simulink model "threephase_transformer"  (R2021a)
settings: Solver=VariableStepAuto  StartTime=0.0  StopTime=0.05  RelTol=1e-3
libraries: spsCurrentMeasurementLib x6, spsVoltageMeasurementLib x6, spsACVoltageSourceLib x3, spsGroundLib x3, spsSeriesRLCBranchLib x3, spsThreePhaseTransformerTwoWindingsLib x1, spspowerguiLib x1
settings Model: Creator=Davie  LastModifiedBy=Davie

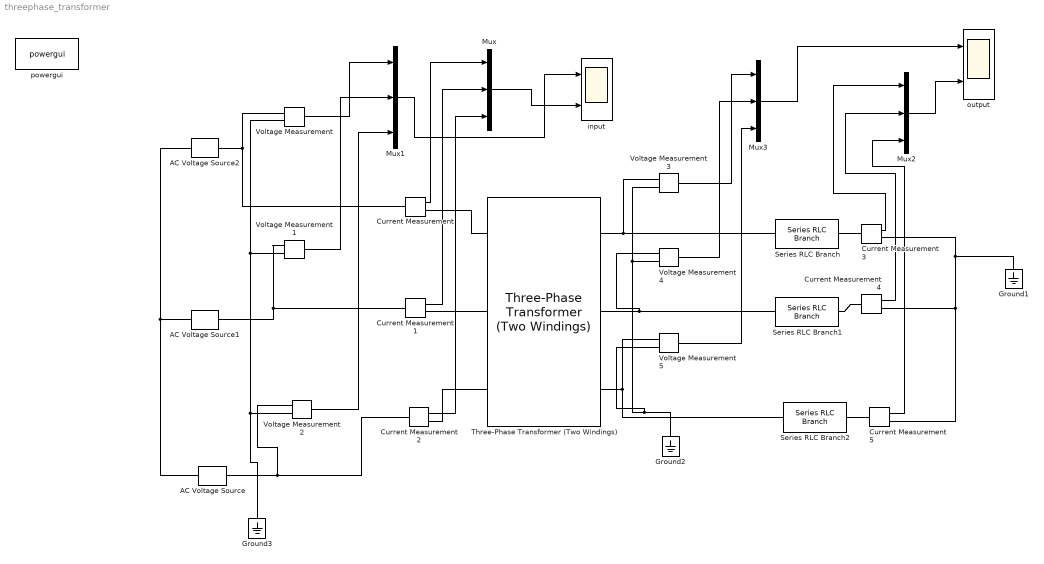
== system threephase_transformer ==
  AC Voltage Source : spsACVoltageSourceLib/AC Voltage Source  Amplitude=450  Phase=-120  Frequency=50  SampleTime=0  Measurements=None  BusType=swing  Pref=10e3  Qref=0  Qmin=-inf  Qmax=+inf
  AC Voltage Source1 : spsACVoltageSourceLib/AC Voltage Source  Amplitude=450  Phase=120  Frequency=50  SampleTime=0  Measurements=None  BusType=swing  Pref=10e3  Qref=0  Qmin=-inf  Qmax=+inf
  AC Voltage Source2 : spsACVoltageSourceLib/AC Voltage Source  Amplitude=450  Phase=0  Frequency=50  SampleTime=0  Measurements=None  BusType=swing  Pref=10e3  Qref=0  Qmin=-inf  Qmax=+inf
  Current Measurement{,1..5} (6 alike) : spsCurrentMeasurementLib/Current Measurement  PhasorSimulation=off  OutputType=Complex  PSBequivalent=0
  Ground1 : spsGroundLib/Ground  LConnTagsString=a
  Ground2 : spsGroundLib/Ground  LConnTagsString=a
  Ground3 : spsGroundLib/Ground  LConnTagsString=a
  Mux{,1..3} (4 alike) : Mux  Inputs=3
  Series RLC Branch : spsSeriesRLCBranchLib/Series RLC Branch  LConnTagsString=__new0  RConnTagsString=__new0  BranchType=R  Resistance=220  Inductance=1e-3  SetiL0=off  InitialCurrent=0  Capacitance=1e-6  Setx0=off  InitialVoltage=0  Measurements=None
  Series RLC Branch1 : spsSeriesRLCBranchLib/Series RLC Branch  LConnTagsString=__new0  RConnTagsString=__new0  BranchType=R  Resistance=220  Inductance=1e-3  SetiL0=off  InitialCurrent=0  Capacitance=1e-6  Setx0=off  InitialVoltage=0  Measurements=None
  Series RLC Branch2 : spsSeriesRLCBranchLib/Series RLC Branch  LConnTagsString=__new0  RConnTagsString=__new0  BranchType=R  Resistance=220  Inductance=1e-3  SetiL0=off  InitialCurrent=0  Capacitance=1e-6  Setx0=off  InitialVoltage=0  Measurements=None
  Three-Phase Transformer (Two Windings) : spsThreePhaseTransformerTwoWindingsLib/Three-Phase Transformer (Two Windings)  Winding1Connection=Yg  Winding2Connection=Yg  CoreType=Three single-phase transformers  SetSaturation=off  Hysteresis=off  DataFile='hysteresis'  SetInitialFlux=off  Measurements=None  UNITS=pu  NominalPower=[ 250e6 , 60 ]  Winding1=[ 440e3 , 0.002 , 0.08 ]  Winding2=[ 315e3 , 0.002 , 0.08 ]  Rm=500  Lm=500  L0=0.5  Saturation=[ 0,0 ; 0.0024,1.2 ; 1.0,1.52 ]  InitialFluxes=[ 0.8 , -0.8 , 0.7 ]  BreakLoop=off  DiscreteSolver=Trapezoidal iterative  DataType=off  TransfoNumber=1
  Voltage Measurement{,1..5} (6 alike) : spsVoltageMeasurementLib/Voltage Measurement  PhasorSimulation=off  OutputType=Complex  PSBequivalent=0
  input : Scope  NumInputPorts=2
  output : Scope  NumInputPorts=2
  powergui : spspowerguiLib/powergui  Priority=1  SimulationMode=Discrete  SampleTime=5e-6  frequency=60  Iterations=50  frequencyindice=50  Pbase=100e6  ErrMax=1e-4  UnitsV=kV  UnitsW=MW  buscounter=0  FunctionMessages=off  echomessages=off  EnableUseOfTLC=off  CurrentSourceSwitches=off  DisableSnubberDevices=off  DisableRonSwitches=off  DisableVfSwitches=off  DisplayEquations=off  AutomaticDiscreteSolvers=off  SolverType=Tustin/Backward Euler (TBE)  Interpol=off  ExternalGateDelay=off  methode=off  Ts=100  x0status=blocks  SPID=on  SwTol=0  HookPort=off  NonlinearTolerance=1e-4  nMaxIteration=100  ContinueOnMaxIteration=off  RestoreLinks=warning  ResistiveCurrentMeasurement=off  Frange=[0:2:500]  Ylog=off  Xlog=on  ShowGrid=off  save=off  variable=ZData  structure=0  ZoomFFT=off  StartTime=0.0  cycles=1  DisplayStyle=1  fundamental=60  FreqAxis=off  MaxFrequency=1000  frequencyindicesteady=1  RmsSteady=1  display=off
  wires:
  Voltage Measurement/1 -> Mux1/1
  Voltage Measurement1/1 -> Mux1/2
  Voltage Measurement2/1 -> Mux1/3
  Current Measurement/1 -> Mux/1
  Current Measurement1/1 -> Mux/2
  Current Measurement2/1 -> Mux/3
  Mux1/1 -> input/1
  Mux/1 -> input/2
  Voltage Measurement3/1 -> Mux3/1
  Voltage Measurement4/1 -> Mux3/2
  Voltage Measurement5/1 -> Mux3/3
  Current Measurement3/1 -> Mux2/1
  Current Measurement4/1 -> Mux2/2
  Current Measurement5/1 -> Mux2/3
  Mux3/1 -> output/1
  Mux2/1 -> output/2
  connections:
  AC Voltage Source2/RConn1 -- Current Measurement/LConn1 -- Voltage Measurement/LConn1
  AC Voltage Source1/RConn1 -- Voltage Measurement1/LConn1 -- Current Measurement1/LConn1
  Voltage Measurement2/LConn1 -- AC Voltage Source/RConn1 -- Current Measurement2/LConn1
  AC Voltage Source2/LConn1 -- AC Voltage Source1/LConn1 -- AC Voltage Source/LConn1
  Current Measurement/RConn1 -- Three-Phase Transformer (Two Windings)/LConn1
  Current Measurement1/RConn1 -- Three-Phase Transformer (Two Windings)/LConn2
  Current Measurement2/RConn1 -- Three-Phase Transformer (Two Windings)/LConn3
  Voltage Measurement3/LConn2 -- Voltage Measurement4/LConn2 -- Voltage Measurement5/LConn2 -- Ground2/LConn1
  Three-Phase Transformer (Two Windings)/RConn2 -- Voltage Measurement4/LConn1 -- Series RLC Branch1/LConn1
  Three-Phase Transformer (Two Windings)/RConn1 -- Voltage Measurement3/LConn1 -- Series RLC Branch/LConn1
  Current Measurement3/LConn1 -- Series RLC Branch/RConn1
  Current Measurement4/LConn1 -- Series RLC Branch1/RConn1
  Current Measurement5/LConn1 -- Series RLC Branch2/RConn1
  Current Measurement3/RConn1 -- Ground1/LConn1 -- Current Measurement4/RConn1 -- Current Measurement5/RConn1
  Three-Phase Transformer (Two Windings)/RConn3 -- Voltage Measurement5/LConn1 -- Series RLC Branch2/LConn1
  Voltage Measurement1/LConn2 -- Voltage Measurement/LConn2 -- Ground3/LConn1 -- Voltage Measurement2/LConn2
